simulink model "HDLConstellationScrambler"  (R2024a)
settings: Solver=FixedStepDiscrete  StartTime=0.0  StopTime=stopTime  RelTol=1e-3
values from neighbouring files (symbols this model uses):
  dataSymbols = [ ... (first row only)    [testConstellationScrambler.m]
undefined symbols (not defined in the file or in its folder): CONST
libraries: hdlsllib x3, dspsrcs4 x2, HDL_ieee_8021513 x2
settings Model: DataTypeOverride=Off  Creator=cotti  LastModifiedBy=cotti
settings OptimizationCC: BlockReduction=off  ConditionallyExecuteInputs=off  DefaultParameterBehavior=Inlined  InheritOutputTypeSmallerThanSingle=on
settings DebuggingCC: AlgebraicLoopMsg=error  ArtificialAlgebraicLoopMsg=error  SingleTaskRateTransMsg=error  UnconnectedInputMsg=warning  UnconnectedOutputMsg=warning  UnconnectedLineMsg=warning
settings HardwareCC: ProdBitPerPointer=32  ProdBitPerSizeT=32  ProdBitPerPtrDiffT=32  ProdLargestAtomicFloat=None  ProdIntDivRoundTo=Undefined  ProdEndianess=Unspecified  ProdWordSize=32  ProdHWDeviceType=ASIC/FPGA->ASIC/FPGA  TargetBitPerLong=64  TargetBitPerPointer=64  TargetBitPerSizeT=64  TargetBitPerPtrDiffT=64  TargetLongLongMode=on  TargetIntDivRoundTo=Zero  TargetEndianess=LittleEndian  TargetWordSize=64  TargetHWDeviceType=Custom Processor->MATLAB Host Computer  ProdEqTarget=off

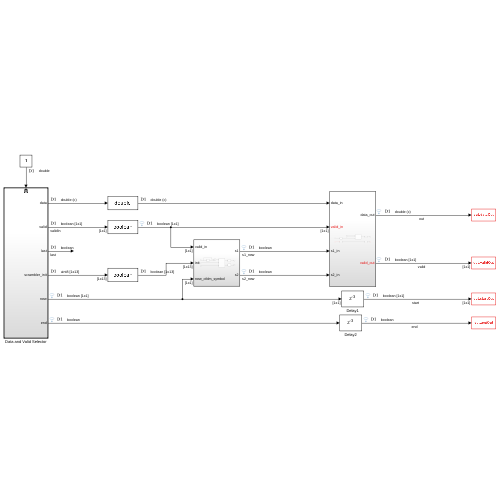
[thumbnail: Simulink's stored preview of the top-level diagram]
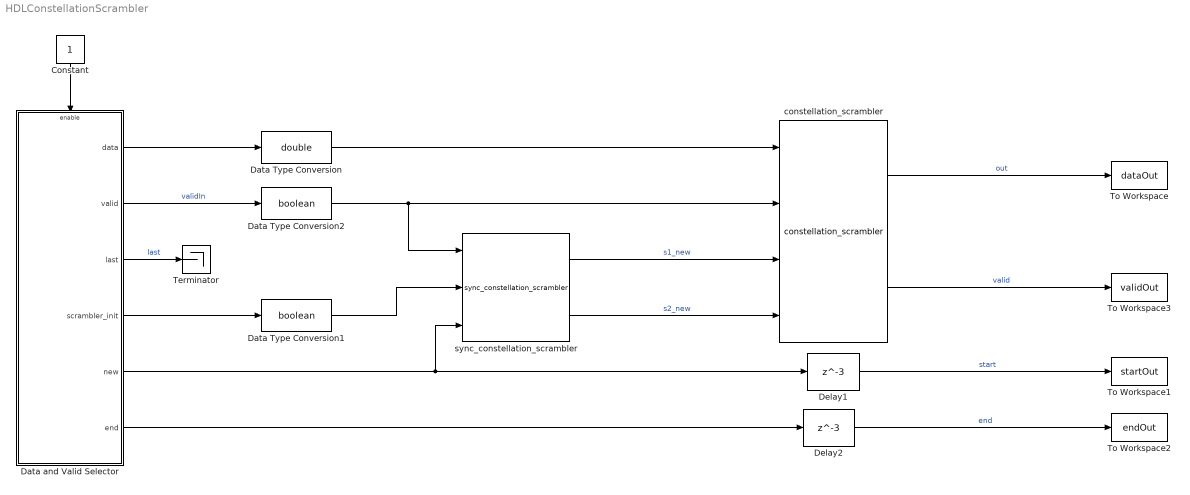
== system HDLConstellationScrambler ==
  Constant : Constant  SampleTime=-1
  Data Type Conversion : DataTypeConversion  OutDataTypeStr=double  SaturateOnIntegerOverflow=off  RndMeth=Floor
  Data Type Conversion1 : DataTypeConversion  OutDataTypeStr=boolean  SaturateOnIntegerOverflow=off  RndMeth=Floor
  Data Type Conversion2 : DataTypeConversion  OutDataTypeStr=boolean  SaturateOnIntegerOverflow=off  RndMeth=Floor
  Data and Valid Selector : Subsystem  TreatAsAtomicUnit=on
  Delay1 : Delay  DelayLength=3  InitialCondition=0  UseCircularBuffer=on
  Delay2 : Delay  DelayLength=3  InitialCondition=0  UseCircularBuffer=on
  Terminator : Terminator
  To Workspace : ToWorkspace  VariableName=dataOut  SampleTime=1/CONST.fPHY
      settings: Save2DSignal=2-D array (concatenate along first dimension)
  To Workspace1 : ToWorkspace  VariableName=startOut  SampleTime=1/CONST.fPHY
      settings: Save2DSignal=2-D array (concatenate along first dimension)
  To Workspace2 : ToWorkspace  VariableName=endOut  SampleTime=1/CONST.fPHY
      settings: Save2DSignal=2-D array (concatenate along first dimension)
  To Workspace3 : ToWorkspace  VariableName=validOut  SampleTime=1/CONST.fPHY
      settings: Save2DSignal=2-D array (concatenate along first dimension)
  constellation_scrambler : HDL_ieee_8021513/constellation_scrambler  SystemSampleTime=-1  VariantActivationTime=update diagram  AllowFlexibleInterface=on  Latency=0  AutoFrameSizeCalculation=off
      settings: SourceProductName=HDL IEEE 8021513
  sync_constellation_scrambler : HDL_ieee_8021513/sync_constellation_scrambler  SystemSampleTime=-1  VariantActivationTime=update diagram  AllowFlexibleInterface=on  Latency=0  AutoFrameSizeCalculation=off
      settings: SourceProductName=HDL IEEE 8021513
  wires:
  Data and Valid Selector/2(valid) -> Data Type Conversion2/1  "validIn"
  Constant/1 -> Data and Valid Selector/Enable
  Data and Valid Selector/1(data) -> Data Type Conversion/1
  constellation_scrambler/2 -> To Workspace3/1  "valid"
  Data and Valid Selector/3(last) -> Terminator/1  "last"
  constellation_scrambler/1 -> To Workspace/1  "out"
  Data and Valid Selector/4(scrambler_init) -> Data Type Conversion1/1
  Data and Valid Selector/5(new) -> Delay1/1, sync_constellation_scrambler/3
  Data and Valid Selector/6(end) -> Delay2/1
  Delay1/1 -> To Workspace1/1  "start"
  Delay2/1 -> To Workspace2/1  "end"
  Data Type Conversion1/1 -> sync_constellation_scrambler/2
  sync_constellation_scrambler/1 -> constellation_scrambler/3  "s1_new"
  sync_constellation_scrambler/2 -> constellation_scrambler/4  "s2_new"
  Data Type Conversion/1 -> constellation_scrambler/1
  Data Type Conversion2/1 -> constellation_scrambler/2, sync_constellation_scrambler/1

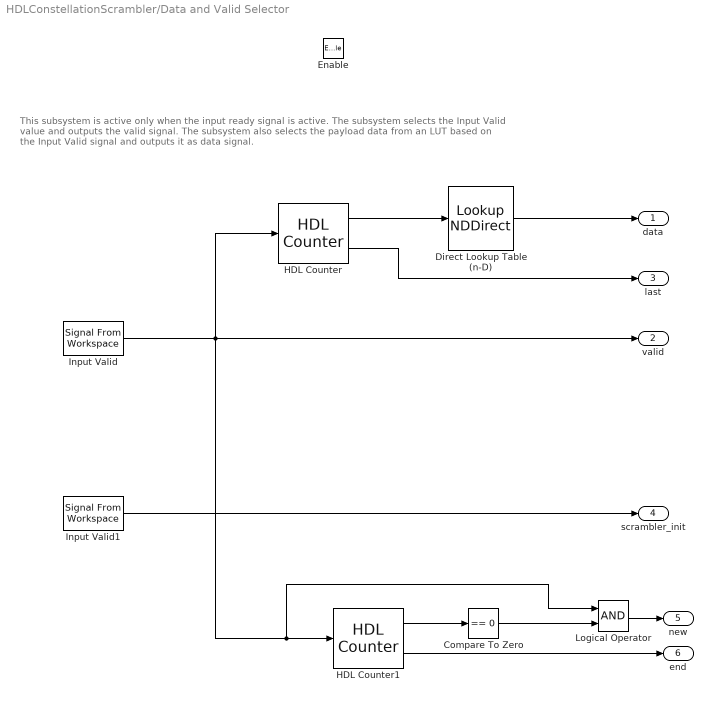
== system HDLConstellationScrambler/Data and Valid Selector ==
  note: This subsystem is active only when the input ready signal is active. The subsystem selects the Input Valid value and outputs the valid signal.
      | The subsystem also selects the payload data from an LUT based on the Input Valid signal and outputs it as data signal.
  Enable : EnablePort
  Compare To Zero : hdlsllib/Logic and Bit Operations/Compare To Zero  relop===  OutDataTypeStr=boolean
  Direct Lookup Table (n-D) : LookupNDDirect  NumberOfTableDimensions=1  Table=dataSymbols  DiagnosticForOutOfRangeInput=Error  TableDataTypeStr=double
  HDL Counter : hdlsllib/Sources/HDL Counter  CountType=Count limited  CountInit=0  CountStep=1  CountMax=length(dataSymbols) -1  CountFromType=Initial value  CountFrom=0  CountResetPort=off  CountLoadPort=off  CountEnbPort=on  CountDirPort=off  CountHitOutputPort=on  CountDataType=Unsigned  CountWordLen=nextpow2(length(dataSymbols))  CountFracLen=0  CountSampTime=1
  HDL Counter1 : hdlsllib/Sources/HDL Counter  CountType=Count limited  CountInit=0  CountStep=1  CountMax=CONST.numDataCarriers-1  CountFromType=Initial value  CountFrom=0  CountResetPort=off  CountLoadPort=off  CountEnbPort=on  CountDirPort=off  CountHitOutputPort=on  CountDataType=Unsigned  CountWordLen=nextpow2(CONST.numDataCarriers)  CountFracLen=0  CountSampTime=1
  Input Valid : dspsrcs4/Signal From Workspace  X=validIn  Ts=1/CONST.fPHY  nsamps=1  OutputAfterFinalValue=Setting to zero  ignoreOrWarnInputAndFrameLengths=off  OutputFrames=off
  Input Valid1 : dspsrcs4/Signal From Workspace  X=scramblerInit  Ts=1/CONST.fPHY  nsamps=1  OutputAfterFinalValue=Setting to zero  ignoreOrWarnInputAndFrameLengths=off  OutputFrames=off
  Logical Operator : Logic  AllPortsSameDT=off  OutDataTypeStr=boolean
  data : Outport  InitialOutput=0  VectorParamsAs1DForOutWhenUnconnected=off
  valid : Outport  Port=2  InitialOutput=0  VectorParamsAs1DForOutWhenUnconnected=off
  last : Outport  Port=3  VectorParamsAs1DForOutWhenUnconnected=off
  scrambler_init : Outport  Port=4  VectorParamsAs1DForOutWhenUnconnected=off
  new : Outport  Port=5  VectorParamsAs1DForOutWhenUnconnected=off
  end : Outport  Port=6  VectorParamsAs1DForOutWhenUnconnected=off
  wires:
  HDL Counter/1 -> Direct Lookup Table (n-D)/1
  Input Valid/1 -> Logical Operator/1, HDL Counter1/1, HDL Counter/1, valid/1
  Direct Lookup Table (n-D)/1 -> data/1
  HDL Counter/2 -> last/1
  Input Valid1/1 -> scrambler_init/1
  HDL Counter1/1 -> Compare To Zero/1
  Compare To Zero/1 -> Logical Operator/2
  Logical Operator/1 -> new/1
  HDL Counter1/2 -> end/1
